simulink model "intSystem"  (R2026a)
settings: Solver=ode3  StopTime=1  FixedStep=xp.Ts
model workspace (MATLAB code in the model file):
  | ip = invParams();
  | wp = windParams();
  | wp = rmfield(wp, {'li_inv','Cp'});   % function handles cannot live on a block
  | xp = intParams();
libraries: fl_lib x17, nesl_utility x15, ee_lib x5, invLib x4, slpidlib x3, windLib x2, simulink x1
settings Model: Creator=khiem  LastModifiedBy=khiem
settings DebuggingCC: AlgebraicLoopMsg=error
settings SimscapeCC: SimscapeLogType=none

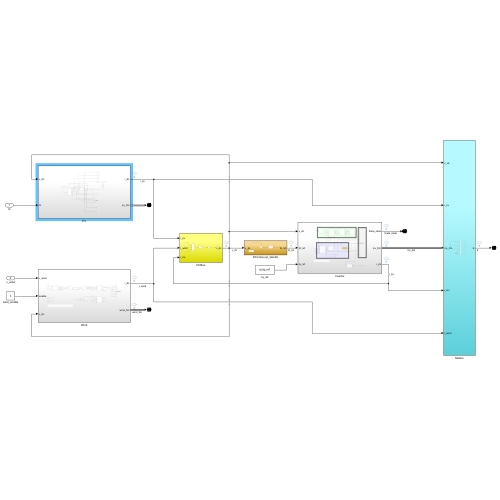
[thumbnail: Simulink's stored preview of the top-level diagram]
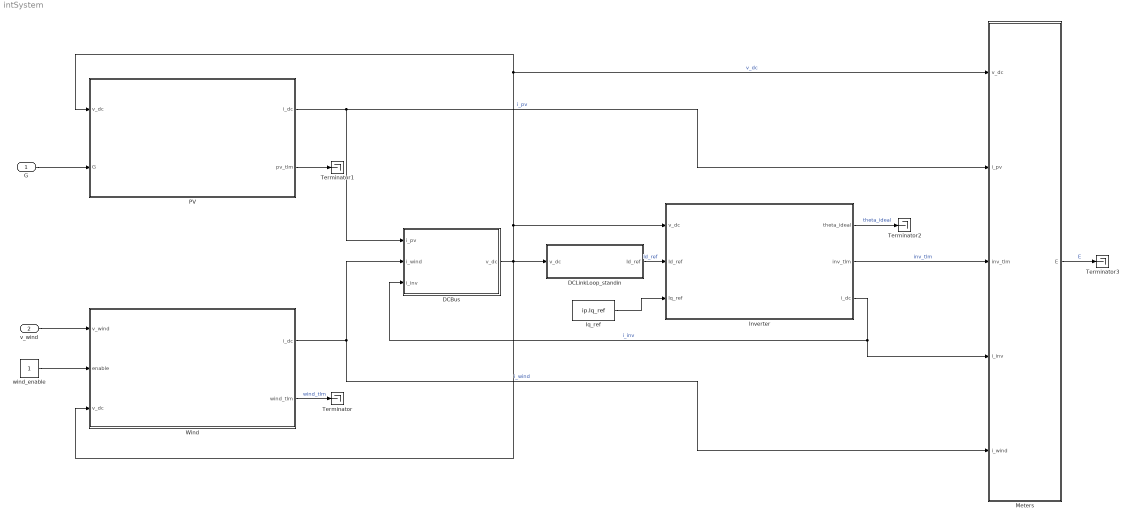
== system intSystem ==
  G : Inport  Interpolate=off
  v_wind : Inport  Port=2  Interpolate=off
  DCBus : Subsystem
  DCLinkLoop_standin : Subsystem
  Inverter : Subsystem
  Iq_ref : Constant  Value=ip.Iq_ref
  Meters : Subsystem
  PV : Subsystem
  Terminator{,1..3} (4 alike) : Terminator
  Wind : Subsystem
  wind_enable : Constant
  wires:
  Inverter/2(inv_tlm) -> Meters/3(inv_tlm)  "inv_tlm"
  G/1 -> PV/2(G)
  v_wind/1 -> Wind/1(v_wind)
  wind_enable/1 -> Wind/2(enable)
  Iq_ref/1 -> Inverter/3(Iq_ref)
  PV/1(i_dc) -> DCBus/1(i_pv), Meters/2(i_pv)  "i_pv"
  Wind/1(i_dc) -> DCBus/2(i_wind), Meters/5(i_wind)  "i_wind"
  Inverter/3(i_dc) -> Meters/4(i_inv), DCBus/3(i_inv)  "i_inv"
  DCBus/1(v_dc) -> Inverter/1(v_dc), Meters/1(v_dc), PV/1(v_dc), DCLinkLoop_standin/1(v_dc), Wind/3(v_dc)  "v_dc"
  DCLinkLoop_standin/1(Id_ref) -> Inverter/2(Id_ref)  "Id_ref"
  Wind/2(wind_tlm) -> Terminator/1  "wind_tlm"
  PV/2(pv_tlm) -> Terminator1/1
  Inverter/1(theta_ideal) -> Terminator2/1  "theta_ideal"
  Meters/1(E) -> Terminator3/1  "E"

== system intSystem/DCBus ==
  i_pv : Inport
  i_wind : Inport  Port=2
  i_inv : Inport  Port=3
  Add : Sum  Inputs=++-
  Gain : Gain  Gain=1/xp.C_bus
  Integrator : Integrator  InitialCondition=xp.Vdc0
  v_dc : Outport
  wires:
  Add/1 -> Gain/1
  Gain/1 -> Integrator/1
  Integrator/1 -> v_dc/1
  i_pv/1 -> Add/1
  i_wind/1 -> Add/2
  i_inv/1 -> Add/3

== system intSystem/DCLinkLoop_standin ==
  v_dc : Inport
  PID Controller : slpidlib/PID Controller  Controller=PI  Form=Parallel  TimeDomain=Discrete-time  UseExternalTs=off  SampleTime=xp.Ts_ctrl  IntegratorMethod=Forward Euler  FilterMethod=Forward Euler  ControllerParametersSource=internal  P=xp.dc.Kp  I=xp.dc.Ki  UseKiTs=off  D=0  UseExternalDerivativeSource=off  N=100  UseFilter=on  TunerSelectOption=Transfer Function Based (PID Tuner App)  InitialConditionSource=internal  InitialConditionForIntegrator=0  InitialConditionForFilter=0  DifferentiatorICPrevScaledInput=0  ExternalReset=none  TrackingMode=off  Kt=1  LimitOutput=on  SatLimitsSource=internal  UpperSaturationLimit=xp.dc.Id_max  LowerSaturationLimit=-xp.dc.Id_max  LinearizeAsGain=on  AntiWindupMode=clamping  Kb=1  LimitIntegrator=off  UpperIntegratorSaturationLimit=inf  LowerIntegratorSaturationLimit=-inf  POutMin=[]  POutMax=[]  IOutMin=[]  IOutMax=[]  DOutMin=[]  DOutMax=[]  NOutMin=[]  NOutMax=[]  SumOutMin=[]  SumOutMax=[]  SaturationOutMin=[]  SaturationOutMax=[]  PParamMin=[]  PParamMax=[]  IParamMin=[]  IParamMax=[]  DParamMin=[]  DParamMax=[]  NParamMin=[]  NParamMax=[]  KbParamMin=[]  KbParamMax=[]  KtParamMin=[]  KtParamMax=[]  KbOutMin=[]  KbOutMax=[]  KtOutMin=[]  KtOutMax=[]  IntegratorOutMin=[]  IntegratorOutMax=[]  FilterOutMin=[]  FilterOutMax=[]  SumI1OutMin=[]  SumI1OutMax=[]  SumI2OutMin=[]  SumI2OutMax=[]  SumI3OutMin=[]  SumI3OutMax=[]  SumI4OutMin=[]  SumI4OutMax=[]  SumDOutMin=[]  SumDOutMax=[]  DifferentiatorOutMin=[]  DifferentiatorOutMax=[]  FilterDiffOutCoefMin=[]  FilterDiffOutCoefMax=[]  ReciprocalOutMin=[]  ReciprocalOutMax=[]  SumDenOutMin=[]  SumDenOutMax=[]  SumNumOutMin=[]  SumNumOutMax=[]  DivideOutMin=[]  DivideOutMax=[]  UdiffTsProdOutMin=[]  UdiffTsProdOutMax=[]  NTsProdOutMin=[]  NTsProdOutMax=[]  UintegralTsProdOutMin=[]  UintegralTsProdOutMax=[]  UngainTsProdOutMin=[]  UngainTsProdOutMax=[]  ClampingZeroOutDataTypeStr=Inherit: Inherit via back propagation  ClampingZeroOutMin=[]  ClampingZeroOutMax=[]  FilterDenConstantOutDataTypeStr=Inherit: Inherit via back propagation  FilterDenConstantOutMin=[]  FilterDenConstantOutMax=[]  PCopyOutDataTypeStr=Inherit: Inherit via back propagation  PCopyOutMin=[]  PCopyOutMax=[]  NCopyOutDataTypeStr=Inherit: Inherit via back propagation  NCopyOutMin=[]  NCopyOutMax=[]  IntegratorContinuousStateAttributes=''  IntegratorStateMustResolveToSignalObject=off  IntegratorRTWStateStorageClass=Auto  FilterContinuousStateAttributes=''  FilterStateMustResolveToSignalObject=off  FilterRTWStateStorageClass=Auto  ParallelPVariant=InternalParameters  IdealPVariant=Disabled  IVariant=InternalParameters  DVariant=Disabled  IntegratorVariant=Discrete  SatVariant=Enabled  AWVariant=DiscClampingParallel  PCopyVariant=Disabled  TRVariant=Disabled  FdbkBlocksVariant=Forward  IdealPFdbkVariant=Disabled  SatFdbkVariant=Disabled  DerivativeFilterVariant=Disabled  NVariant=Disabled  NCopyVariant=Disabled_SignalSpec  FilterICVariant=Disabled  IntegratorICVariant=InternalICs  ExternalResetVariant=Disabled  TRSumVariant=Passthrough  SumFdbkVariant=Disabled  SumVariant=Sum_PI  TsampFilterVariant=InternalTs  TsampNgainVariant=Passthrough  TsampIntegralVariant=Disabled_SignalSpec  ExternalSaturationOutDataTypeStr=Inherit: Same as second input  DerivativeSourceVariant=Disabled  PreIntVariant=InternalPreInt
  Sum : Sum  Inputs=+-
  Vdc_ref : Constant  Value=xp.Vdc_ref
  Id_ref : Outport
  wires:
  v_dc/1 -> Sum/1
  PID Controller/1 -> Id_ref/1
  Sum/1 -> PID Controller/1
  Vdc_ref/1 -> Sum/2

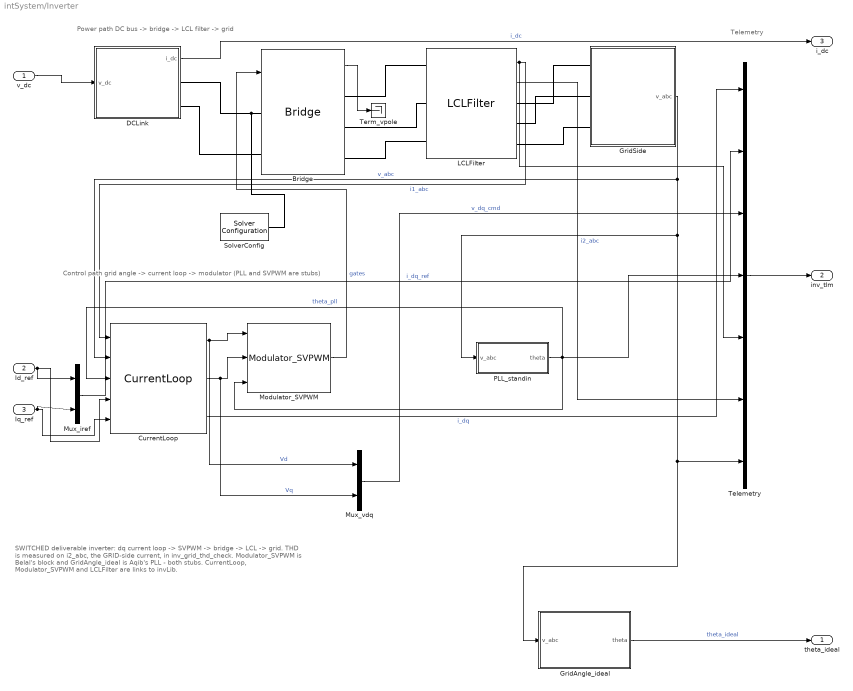
== system intSystem/Inverter ==
  note: SWITCHED deliverable inverter: dq current loop -> SVPWM -> bridge -> LCL -> grid.
      | THD is measured on i2_abc, the GRID-side current, in inv_grid_thd_check.
      | Modulator_SVPWM is Belal's block and GridAngle_ideal is Aqib's PLL - both stubs.
      | CurrentLoop, Modulator_SVPWM and LCLFilter are links to invLib.
  note: Power path DC bus -> bridge -> LCL filter -> grid
  note: Telemetry
  note: Control path grid angle -> current loop -> modulator (PLL and SVPWM are stubs)
  v_dc : Inport
  Id_ref : Inport  Port=2
  Iq_ref : Inport  Port=3
  Bridge : invLib/Bridge  SystemSampleTime=-1  VariantActivationTime=update diagram  EmptyChoice=off  PassThrough=off  PassThroughVariantControl=(default)  EmptyChoiceVariantControl=(default)  AllowFlexibleInterface=on  Latency=0  AutoFrameSizeCalculation=off
  CurrentLoop : invLib/CurrentLoop  SystemSampleTime=-1  VariantActivationTime=update diagram  EmptyChoice=off  PassThrough=off  PassThroughVariantControl=(default)  EmptyChoiceVariantControl=(default)  AllowFlexibleInterface=on  Latency=0  AutoFrameSizeCalculation=off
  DCLink : Subsystem
  GridAngle_ideal : Subsystem
  GridSide : Subsystem
  LCLFilter : invLib/LCLFilter  SystemSampleTime=-1  VariantActivationTime=update diagram  EmptyChoice=off  PassThrough=off  PassThroughVariantControl=(default)  EmptyChoiceVariantControl=(default)  AllowFlexibleInterface=on  Latency=0  AutoFrameSizeCalculation=off
  Modulator_SVPWM : invLib/Modulator_SVPWM  SystemSampleTime=-1  VariantActivationTime=update diagram  EmptyChoice=off  PassThrough=off  PassThroughVariantControl=(default)  EmptyChoiceVariantControl=(default)  AllowFlexibleInterface=on  Latency=0  AutoFrameSizeCalculation=off
  Mux_iref : Mux  Inputs=2
  Mux_vdq : Mux  Inputs=2
  PLL_standin : Subsystem
  SolverConfig : nesl_utility/Solver Configuration  PhysicalDomain=network_engine_domain  SubClassName=solver  LeftPortType=input  RightPortType=generic  Tones=[]  Harmonics=[]  SimulateNoise=off  Profile=off  UseLocalSampling=off  EnableSwitchedLinearOptims=on  FrequencyDomain=off  UseCCode=off  RelTol=0.001  AbsTol=0.001  MinStep=1e-09  ToWorkspace=off  RevertToSquareIcSolve=off  NumHomotopyIterations=100  PhasorMode=off  PhasorModeNumHarmonics=1  ConsistencySolver=NEWTON_XTOL_AFTER_FTOL  CanonicalOrdering=CANONICAL  OptimizeIntermediates=OPTIMIZED  IndexReductionMethod=DerivativeReplacement  DoDC=off  ResidualTolerance=1e-09  ConsistencyTolSource=GLOBAL  ConsistencyAbsTol=0.001  ConsistencyRelTol=0.001  ConsistencyTolFactor=0.001  UseLocalSolver=on  LocalSolverChoice=NE_BACKWARD_EULER_ADVANCER  ResolveIndetEquations=on  FunctionEvalNumThread=1  LocalSolverSampleTime=ip.Ts_power  DoFixedCost=off  MaxNonlinIter=3  MaxModeIter=2  ComputeImpulses=off  ImpulseIterations=2  LinearAlgebra=auto  LinearAlgebraNumThread=0  EquationFormulation=NE_TIME_EF  DelaysMemoryBudget=1024  AutomaticFiltering=on  FilteringTimeConstant=0.001  PartitionStorageMethod=AS_NEEDED  PartitionMemoryBudget=1024  PartitionMethod=ROBUST  MultibodyUseLocalSolver=off  MultibodyLocalSolverChoice=ODE1  MultibodyLocalSolverSampleTime=0.001
  Telemetry : BusCreator  Inputs=7
  Term_vpole : Terminator
  theta_ideal : Outport
  inv_tlm : Outport  Port=2
  i_dc : Outport  Port=3
  wires:
  Bridge/1 -> Term_vpole/1
  GridSide/1(v_abc) -> PLL_standin/1(v_abc), GridAngle_ideal/1(v_abc), Telemetry/7, CurrentLoop/2  "v_abc"
  Mux_iref/1 -> Telemetry/2  "i_dq_ref"
  CurrentLoop/3 -> Telemetry/1  "i_dq"
  CurrentLoop/1 -> Modulator_SVPWM/1, Mux_vdq/1  "Vd"
  CurrentLoop/2 -> Modulator_SVPWM/2, Mux_vdq/2  "Vq"
  Modulator_SVPWM/1 -> Bridge/1  "gates"
  LCLFilter/1 -> CurrentLoop/1, Telemetry/5  "i1_abc"
  Id_ref/1 -> CurrentLoop/4, Mux_iref/1
  Iq_ref/1 -> CurrentLoop/5, Mux_iref/2
  DCLink/1(i_dc) -> i_dc/1  "i_dc"
  Telemetry/1 -> inv_tlm/1
  Mux_vdq/1 -> Telemetry/3  "v_dq_cmd"
  v_dc/1 -> DCLink/1(v_dc)
  LCLFilter/2 -> Telemetry/6  "i2_abc"
  PLL_standin/1(theta) -> CurrentLoop/3, Telemetry/4, Modulator_SVPWM/3  "theta_pll"
  GridAngle_ideal/1(theta) -> theta_ideal/1  "theta_ideal"
  connections:
  SolverConfig/RConn1 -- Bridge/LConn1 -- DCLink/RConn1
  Bridge/RConn3 -- LCLFilter/LConn3
  Bridge/RConn1 -- LCLFilter/LConn1
  LCLFilter/RConn1 -- GridSide/LConn1
  Bridge/RConn2 -- LCLFilter/LConn2
  LCLFilter/RConn3 -- GridSide/LConn3
  DCLink/RConn2 -- Bridge/LConn2
  LCLFilter/RConn2 -- GridSide/LConn2

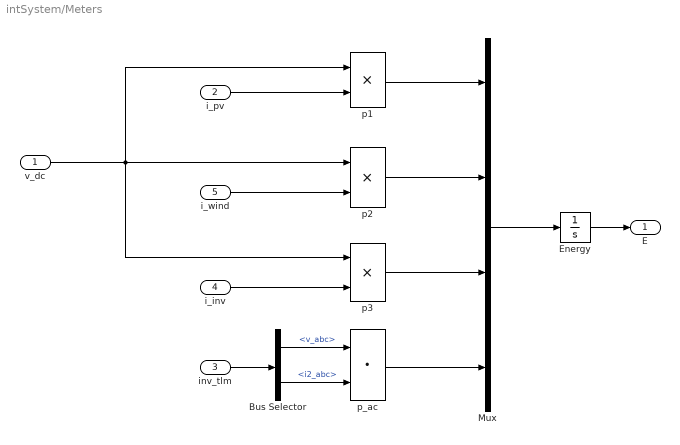
== system intSystem/Meters ==
  v_dc : Inport
  i_pv : Inport  Port=2
  inv_tlm : Inport  Port=3
  i_inv : Inport  Port=4
  i_wind : Inport  Port=5
  Bus Selector : BusSelector  OutputSignals=v_abc,i2_abc
  Energy : Integrator
  Mux : Mux
  p1 : Product
  p2 : Product
  p3 : Product
  p_ac : DotProduct  OutDataTypeStr=Inherit: Inherit via internal rule
  E : Outport
  wires:
  Energy/1 -> E/1
  v_dc/1 -> p3/1, p2/1, p1/1
  i_pv/1 -> p1/2
  i_wind/1 -> p2/2
  i_inv/1 -> p3/2
  p1/1 -> Mux/1
  p2/1 -> Mux/2
  p3/1 -> Mux/3
  inv_tlm/1 -> Bus Selector/1
  Bus Selector/1 -> p_ac/1  "<v_abc>"
  Bus Selector/2 -> p_ac/2  "<i2_abc>"
  p_ac/1 -> Mux/4
  Mux/1 -> Energy/1

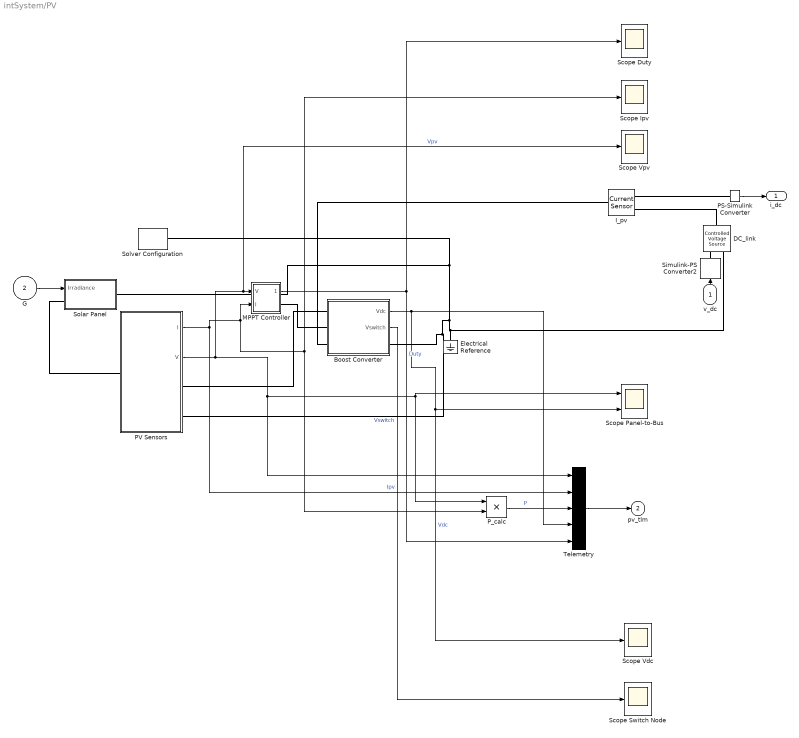
== system intSystem/PV ==
  v_dc : Inport
  G : Inport  Port=2
  Boost Converter : Subsystem
  DC_link : fl_lib/Electrical/Electrical Sources/Controlled Voltage Source
  Electrical Reference : fl_lib/Electrical/Electrical Elements/Electrical Reference
  I_pv : fl_lib/Electrical/Electrical Sensors/Current Sensor
  MPPT Controller : Subsystem
  PS-Simulink Converter : nesl_utility/PS-Simulink Converter  PhysicalDomain=network_engine_domain  SubClassName=ps_output  LeftPortType=input  RightPortType=output  PseudoPeriodic=off  Frequencies=[]  VectorFormat=inherit  Unit=inherit  AffineConversion=off
  PV Sensors : Subsystem
  P_calc : Product
  Scope Duty : Scope
      settings: ActiveDisplayYMinimum=0  ActiveDisplayYMaximum=1
  Scope Ipv : Scope
      settings: ActiveDisplayYMinimum=-14.400000000000034  ActiveDisplayYMaximum=363.59999999999997  DataLoggingVariableName=ScopeData2
  Scope Panel-to-Bus : Scope  NumInputPorts=2
      settings: ActiveDisplayYMinimum=83.437432046539357  ActiveDisplayYMaximum=741.599411880045  DataLoggingVariableName=ScopeData3
  Scope Switch Node : Scope
      settings: ActiveDisplayYMinimum=0  ActiveDisplayYMaximum=800  DataLoggingVariableName=ScopeData4
  Scope Vdc : Scope
      settings: ActiveDisplayYMinimum=551.00007250796614  ActiveDisplayYMaximum=792.77452483583806  DataLoggingVariableName=ScopeData5
  Scope Vpv : Scope
      settings: ActiveDisplayYMinimum=-836.38107028754  ActiveDisplayYMaximum=1247.3439297124605
  Simulink-PS Converter2 : nesl_utility/Simulink-PS Converter  PhysicalDomain=network_engine_domain  SubClassName=ps_input  LeftPortType=input  RightPortType=output  PseudoPeriodic=off  Frequencies=[]  NoiseDistribution=none  NoiseParameters=[]  Unit=1  AffineConversion=off  FilteringAndDerivatives=filter  SimscapeFilterOrder=2  InputFilterTimeConstant=1e-4  UdotUserProvided=0
  Solar Panel : Subsystem  mask(PV Panel){CellTempC=25}
      mask prompts: CellTempC "Cell Temperature (degC)"
      mask help: PV array (5S/48P scaled cell array). Temperature is a per-run parameter, not a live signal -- this Solar Cell block variant has no thermal port (confirmed: no H-port exists), so T_cell cannot vary continuously during one simulation. Set it here before each run.
  Solver Configuration : nesl_utility/Solver Configuration  PhysicalDomain=network_engine_domain  SubClassName=solver  LeftPortType=input  RightPortType=generic  Tones=[]  Harmonics=[]  SimulateNoise=off  Profile=off  UseLocalSampling=off  EnableSwitchedLinearOptims=on  FrequencyDomain=off  UseCCode=off  RelTol=0.001  AbsTol=0.001  MinStep=1e-09  ToWorkspace=off  RevertToSquareIcSolve=off  NumHomotopyIterations=100  PhasorMode=off  PhasorModeNumHarmonics=1  ConsistencySolver=NEWTON_XTOL_AFTER_FTOL  CanonicalOrdering=CANONICAL  OptimizeIntermediates=OPTIMIZED  IndexReductionMethod=DerivativeReplacement  DoDC=off  ResidualTolerance=1e-09  ConsistencyTolSource=GLOBAL  ConsistencyAbsTol=0.001  ConsistencyRelTol=0.001  ConsistencyTolFactor=0.001  UseLocalSolver=on  LocalSolverChoice=NE_BACKWARD_EULER_ADVANCER  ResolveIndetEquations=on  FunctionEvalNumThread=1  LocalSolverSampleTime=xp.Ts  DoFixedCost=off  MaxNonlinIter=3  MaxModeIter=2  ComputeImpulses=off  ImpulseIterations=2  LinearAlgebra=auto  LinearAlgebraNumThread=0  EquationFormulation=NE_TIME_EF  DelaysMemoryBudget=1024  AutomaticFiltering=on  FilteringTimeConstant=0.001  PartitionStorageMethod=AS_NEEDED  PartitionMemoryBudget=1024  PartitionMethod=ROBUST  MultibodyUseLocalSolver=off  MultibodyLocalSolverChoice=ODE1  MultibodyLocalSolverSampleTime=0.001
  Telemetry : BusCreator  Inputs=5
  i_dc : Outport
  pv_tlm : Outport  Port=2
  wires:
  v_dc/1 -> Simulink-PS Converter2/1
  PV Sensors/1(I) -> MPPT Controller/2(I), P_calc/2, Scope Ipv/1, Telemetry/2  "Ipv"
  Boost Converter/2(Vswitch) -> Scope Switch Node/1  "Vswitch"
  MPPT Controller/1(Duty) -> Scope Duty/1, Telemetry/5  "Duty"
  PV Sensors/2(V) -> Telemetry/1, P_calc/1, Scope Panel-to-Bus/1, Scope Vpv/1, MPPT Controller/1(V)  "Vpv"
  G/1 -> Solar Panel/1(Irradiance)
  Boost Converter/1(Vdc) -> Telemetry/4, Scope Vdc/1, Scope Panel-to-Bus/2  "Vdc"
  Telemetry/1 -> pv_tlm/1
  P_calc/1 -> Telemetry/3  "P"
  PS-Simulink Converter/1 -> i_dc/1
  connections:
  PV Sensors/RConn2 -- Boost Converter/RConn1 -- Solver Configuration/RConn1 -- Solar Panel/RConn1 -- DC_link/RConn2 -- Electrical Reference/LConn1
  MPPT Controller/RConn1 -- Boost Converter/LConn2
  PV Sensors/RConn1 -- Boost Converter/LConn1
  Solar Panel/LConn1 -- PV Sensors/LConn1
  Simulink-PS Converter2/RConn1 -- DC_link/RConn1
  Boost Converter/LConn3 -- I_pv/LConn1
  I_pv/RConn2 -- DC_link/LConn1
  I_pv/RConn1 -- PS-Simulink Converter/LConn1

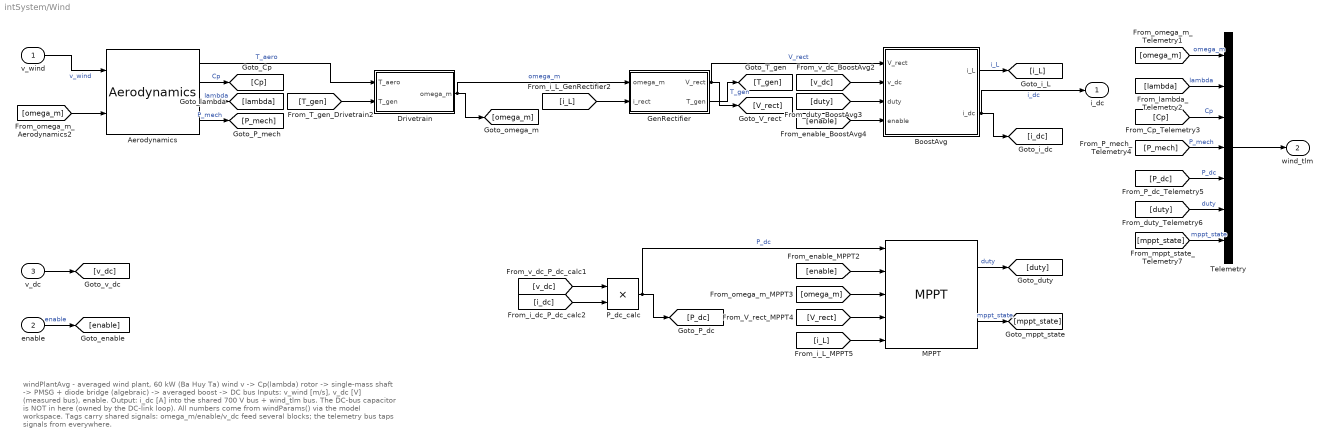
== system intSystem/Wind ==
  note: windPlantAvg - averaged wind plant, 60 kW (Ba Huy Ta)
      | wind v -> Cp(lambda) rotor -> single-mass shaft -> PMSG + diode bridge (algebraic) -> averaged boost -> DC bus
      | Inputs: v_wind [m/s], v_dc [V] (measured bus), enable.  Output: i_dc [A] into the shared 700 V bus + wind_tlm bus.
      | The DC-bus capacitor is NOT in here (owned by the DC-link loop). All numbers come from windParams() via the model workspace.
      | Tags carry shared signals: omega_m/enable/v_dc feed several blocks; the telemetry bus taps signals from everywhere.
  v_wind : Inport
  enable : Inport  Port=2
  v_dc : Inport  Port=3
  Aerodynamics : windLib/Aerodynamics  SystemSampleTime=-1  VariantActivationTime=update diagram  EmptyChoice=off  PassThrough=off  PassThroughVariantControl=(default)  EmptyChoiceVariantControl=(default)  AllowFlexibleInterface=on  Latency=0  AutoFrameSizeCalculation=off
  BoostAvg : Subsystem
  Drivetrain : Subsystem
  GenRectifier : Subsystem
  MPPT : windLib/MPPT  SystemSampleTime=-1  VariantActivationTime=update diagram  EmptyChoice=off  PassThrough=off  PassThroughVariantControl=(default)  EmptyChoiceVariantControl=(default)  AllowFlexibleInterface=on  Latency=0  AutoFrameSizeCalculation=off
  P_dc_calc : Product
  Telemetry : BusCreator  Inputs=7
  i_dc : Outport
  wind_tlm : Outport  Port=2
  wires:
  [omega_m] -> Aerodynamics/2
  [v_dc] -> BoostAvg/2(v_dc)
  [i_dc] -> P_dc_calc/2
  [T_gen] -> Drivetrain/2(T_gen)
  [i_L] -> GenRectifier/2(i_rect)
  Aerodynamics/2 -> [Cp]  "Cp"
  GenRectifier/1(V_rect) -> [V_rect], BoostAvg/1(V_rect)  "V_rect"
  Aerodynamics/4 -> [P_mech]  "P_mech"
  enable/1 -> [enable]  "enable"
  MPPT/1 -> [duty]  "duty"
  Aerodynamics/3 -> [lambda]  "lambda"
  Drivetrain/1(omega_m) -> [omega_m], GenRectifier/1(omega_m)  "omega_m"
  [mppt_state] -> Telemetry/7  "mppt_state"
  Aerodynamics/1 -> Drivetrain/1(T_aero)  "T_aero"
  [P_mech] -> Telemetry/4  "P_mech"
  [v_dc] -> P_dc_calc/1
  [duty] -> BoostAvg/3(duty)
  GenRectifier/2(T_gen) -> [T_gen]  "T_gen"
  v_dc/1 -> [v_dc]
  [enable] -> BoostAvg/4(enable)
  Telemetry/1 -> wind_tlm/1
  [duty] -> Telemetry/6  "duty"
  [enable] -> MPPT/2
  [omega_m] -> MPPT/3
  [Cp] -> Telemetry/3  "Cp"
  [omega_m] -> Telemetry/1  "omega_m"
  [lambda] -> Telemetry/2  "lambda"
  [V_rect] -> MPPT/4
  P_dc_calc/1 -> [P_dc], MPPT/1  "P_dc"
  [i_L] -> MPPT/5
  MPPT/2 -> [mppt_state]  "mppt_state"
  [P_dc] -> Telemetry/5  "P_dc"
  BoostAvg/2(i_dc) -> [i_dc], i_dc/1  "i_dc"
  v_wind/1 -> Aerodynamics/1  "v_wind"
  BoostAvg/1(i_L) -> [i_L]  "i_L"

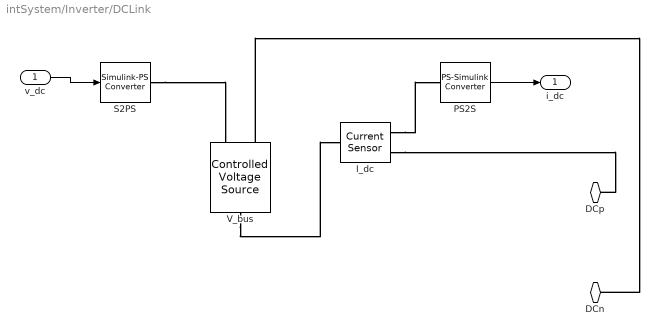
== system intSystem/Inverter/DCLink ==
  v_dc : Inport
  I_dc : fl_lib/Electrical/Electrical Sensors/Current Sensor
  PS2S : nesl_utility/PS-Simulink Converter  PhysicalDomain=network_engine_domain  SubClassName=ps_output  LeftPortType=input  RightPortType=output  PseudoPeriodic=off  Frequencies=[]  VectorFormat=inherit  Unit=inherit  AffineConversion=off
  S2PS : nesl_utility/Simulink-PS Converter  PhysicalDomain=network_engine_domain  SubClassName=ps_input  LeftPortType=input  RightPortType=output  PseudoPeriodic=off  Frequencies=[]  NoiseDistribution=none  NoiseParameters=[]  Unit=1  AffineConversion=off  FilteringAndDerivatives=provide  SimscapeFilterOrder=1  InputFilterTimeConstant=0.001  UdotUserProvided=0
  V_bus : fl_lib/Electrical/Electrical Sources/Controlled Voltage Source
  DCp : PMIOPort  Side=Right
  DCn : PMIOPort  Port=2  Side=Right
  i_dc : Outport
  wires:
  v_dc/1 -> S2PS/1
  PS2S/1 -> i_dc/1
  connections:
  S2PS/RConn1 -- V_bus/RConn1
  V_bus/LConn1 -- I_dc/LConn1
  I_dc/RConn2 -- DCp/RConn1
  V_bus/RConn2 -- DCn/RConn1
  I_dc/RConn1 -- PS2S/LConn1

== system intSystem/Inverter/GridAngle_ideal ==
  v_abc : Inport
  grid_angle : MATLAB Function  TreatAsAtomicUnit=on
  sample_theta : UnitDelay  SampleTime=ip.Ts_ctrl
  theta : Outport
  wires:
  v_abc/1 -> grid_angle/1(v_abc)
  grid_angle/1(theta) -> sample_theta/1
  sample_theta/1 -> theta/1

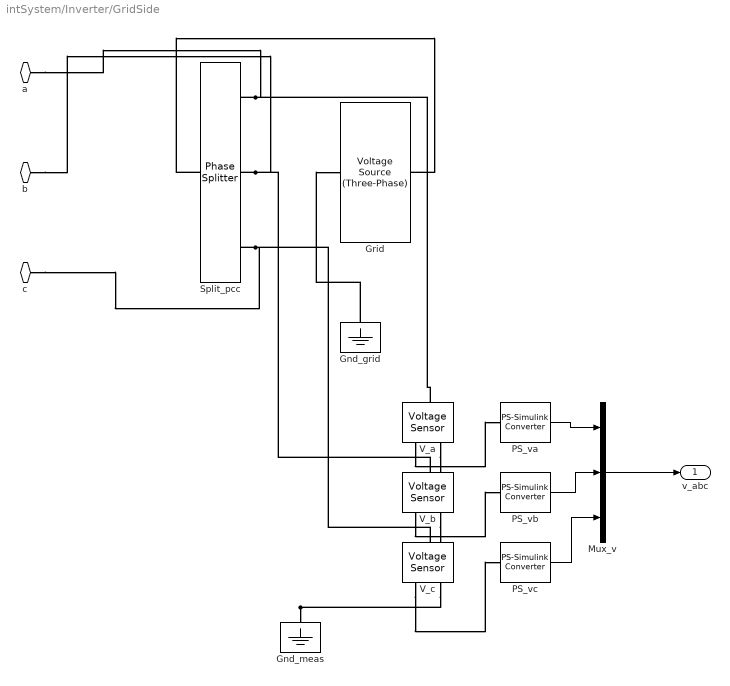
== system intSystem/Inverter/GridSide ==
  Gnd_grid : fl_lib/Electrical/Electrical Elements/Electrical Reference
  Gnd_meas : fl_lib/Electrical/Electrical Elements/Electrical Reference
  Grid : ee_lib/Sources/Voltage Source (Three-Phase)  vline_rms=ip.V_ll V  shift=0 deg  freq=ip.f_grid Hz  impedance_option=ip.grid_Z_opt  SShortCircuit=ip.S_sc A*V  XR=ip.grid_XR  R=0.01 Ohm  L=3.97e-4 H  harmonic_option=0  harmonic_orders=[5, 7, 11, 13]  harmonic_ratios=[.1, .1, .1, .1]  G_parasitic=0 1/Ohm  I_specify=off  I_priority=None  I=[0, 0, 0] A  I_nominal_specify=off  I_nominal_value=1  I_nominal_unit=A
  Mux_v : Mux  Inputs=3
  PS_va : nesl_utility/PS-Simulink Converter  PhysicalDomain=network_engine_domain  SubClassName=ps_output  LeftPortType=input  RightPortType=output  PseudoPeriodic=off  Frequencies=[]  VectorFormat=inherit  Unit=inherit  AffineConversion=off
  PS_vb : nesl_utility/PS-Simulink Converter  PhysicalDomain=network_engine_domain  SubClassName=ps_output  LeftPortType=input  RightPortType=output  PseudoPeriodic=off  Frequencies=[]  VectorFormat=inherit  Unit=inherit  AffineConversion=off
  PS_vc : nesl_utility/PS-Simulink Converter  PhysicalDomain=network_engine_domain  SubClassName=ps_output  LeftPortType=input  RightPortType=output  PseudoPeriodic=off  Frequencies=[]  VectorFormat=inherit  Unit=inherit  AffineConversion=off
  Split_pcc : ee_lib/Connectors & References/Phase Splitter
  V_a : fl_lib/Electrical/Electrical Sensors/Voltage Sensor
  V_b : fl_lib/Electrical/Electrical Sensors/Voltage Sensor
  V_c : fl_lib/Electrical/Electrical Sensors/Voltage Sensor
  a : PMIOPort  Side=Left
  b : PMIOPort  Port=2  Side=Left
  c : PMIOPort  Port=3  Side=Left
  v_abc : Outport
  wires:
  PS_va/1 -> Mux_v/1
  PS_vb/1 -> Mux_v/2
  PS_vc/1 -> Mux_v/3
  Mux_v/1 -> v_abc/1
  connections:
  Split_pcc/LConn1 -- Grid/RConn1
  Gnd_grid/LConn1 -- Grid/LConn1
  Split_pcc/RConn1 -- a/RConn1 -- V_a/LConn1
  V_a/RConn2 -- V_b/RConn2 -- Gnd_meas/LConn1 -- V_c/RConn2
  V_a/RConn1 -- PS_va/LConn1
  Split_pcc/RConn2 -- b/RConn1 -- V_b/LConn1
  V_b/RConn1 -- PS_vb/LConn1
  Split_pcc/RConn3 -- c/RConn1 -- V_c/LConn1
  V_c/RConn1 -- PS_vc/LConn1

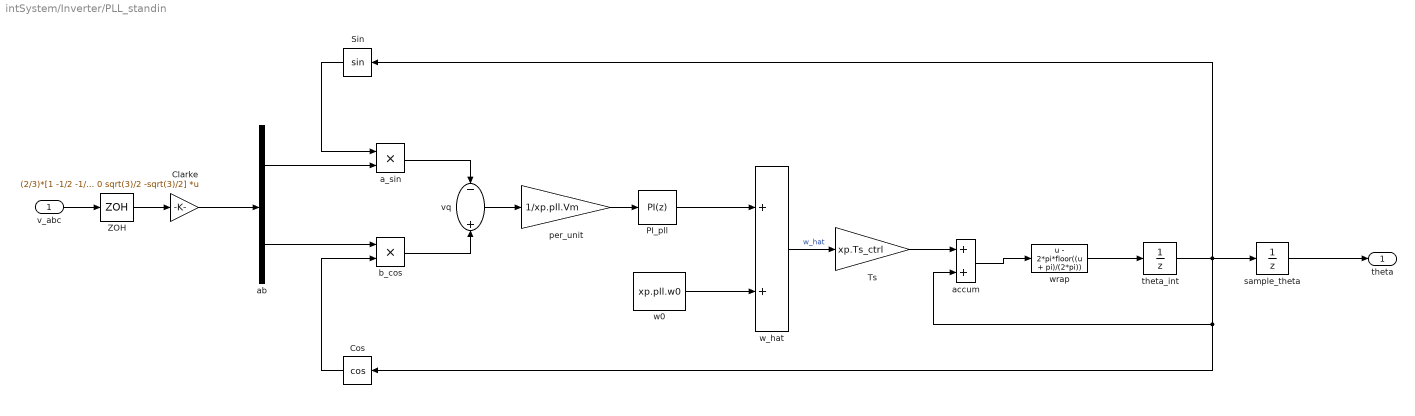
== system intSystem/Inverter/PLL_standin ==
  v_abc : Inport
  " Ts" : Gain  Gain=xp.Ts_ctrl
  " w_hat" : Sum
  Clarke : Gain  Gain=(2/3)*[1 -1/2 -1/2; 0 sqrt(3)/2 -sqrt(3)/2]  Multiplication=Matrix(K*u)
  Cos : Trigonometry  Operator=cos
  PI_pll : slpidlib/PID Controller  Controller=PI  Form=Parallel  TimeDomain=Discrete-time  UseExternalTs=off  SampleTime=xp.Ts_ctrl  IntegratorMethod=Forward Euler  FilterMethod=Forward Euler  ControllerParametersSource=internal  P=xp.pll.Kp  I=xp.pll.Ki  UseKiTs=off  D=0  UseExternalDerivativeSource=off  N=100  UseFilter=on  TunerSelectOption=Transfer Function Based (PID Tuner App)  InitialConditionSource=internal  InitialConditionForIntegrator=0  InitialConditionForFilter=0  DifferentiatorICPrevScaledInput=0  ExternalReset=none  TrackingMode=off  Kt=1  LimitOutput=off  SatLimitsSource=internal  UpperSaturationLimit=inf  LowerSaturationLimit=-inf  LinearizeAsGain=on  AntiWindupMode=none  Kb=1  LimitIntegrator=off  UpperIntegratorSaturationLimit=inf  LowerIntegratorSaturationLimit=-inf  POutMin=[]  POutMax=[]  IOutMin=[]  IOutMax=[]  DOutMin=[]  DOutMax=[]  NOutMin=[]  NOutMax=[]  SumOutMin=[]  SumOutMax=[]  SaturationOutMin=[]  SaturationOutMax=[]  PParamMin=[]  PParamMax=[]  IParamMin=[]  IParamMax=[]  DParamMin=[]  DParamMax=[]  NParamMin=[]  NParamMax=[]  KbParamMin=[]  KbParamMax=[]  KtParamMin=[]  KtParamMax=[]  KbOutMin=[]  KbOutMax=[]  KtOutMin=[]  KtOutMax=[]  IntegratorOutMin=[]  IntegratorOutMax=[]  FilterOutMin=[]  FilterOutMax=[]  SumI1OutMin=[]  SumI1OutMax=[]  SumI2OutMin=[]  SumI2OutMax=[]  SumI3OutMin=[]  SumI3OutMax=[]  SumI4OutMin=[]  SumI4OutMax=[]  SumDOutMin=[]  SumDOutMax=[]  DifferentiatorOutMin=[]  DifferentiatorOutMax=[]  FilterDiffOutCoefMin=[]  FilterDiffOutCoefMax=[]  ReciprocalOutMin=[]  ReciprocalOutMax=[]  SumDenOutMin=[]  SumDenOutMax=[]  SumNumOutMin=[]  SumNumOutMax=[]  DivideOutMin=[]  DivideOutMax=[]  UdiffTsProdOutMin=[]  UdiffTsProdOutMax=[]  NTsProdOutMin=[]  NTsProdOutMax=[]  UintegralTsProdOutMin=[]  UintegralTsProdOutMax=[]  UngainTsProdOutMin=[]  UngainTsProdOutMax=[]  ClampingZeroOutDataTypeStr=Inherit: Inherit via back propagation  ClampingZeroOutMin=[]  ClampingZeroOutMax=[]  FilterDenConstantOutDataTypeStr=Inherit: Inherit via back propagation  FilterDenConstantOutMin=[]  FilterDenConstantOutMax=[]  PCopyOutDataTypeStr=Inherit: Inherit via back propagation  PCopyOutMin=[]  PCopyOutMax=[]  NCopyOutDataTypeStr=Inherit: Inherit via back propagation  NCopyOutMin=[]  NCopyOutMax=[]  IntegratorContinuousStateAttributes=''  IntegratorStateMustResolveToSignalObject=off  IntegratorRTWStateStorageClass=Auto  FilterContinuousStateAttributes=''  FilterStateMustResolveToSignalObject=off  FilterRTWStateStorageClass=Auto  ParallelPVariant=InternalParameters  IdealPVariant=Disabled  IVariant=InternalParameters  DVariant=Disabled  IntegratorVariant=Discrete  SatVariant=Disabled  AWVariant=Passthrough  PCopyVariant=Disabled  TRVariant=Disabled  FdbkBlocksVariant=Forward  IdealPFdbkVariant=Disabled  SatFdbkVariant=Disabled  DerivativeFilterVariant=Disabled  NVariant=Disabled  NCopyVariant=Disabled_SignalSpec  FilterICVariant=Disabled  IntegratorICVariant=InternalICs  ExternalResetVariant=Disabled  TRSumVariant=Passthrough  SumFdbkVariant=Disabled  SumVariant=Sum_PI  TsampFilterVariant=InternalTs  TsampNgainVariant=Passthrough  TsampIntegralVariant=Disabled_SignalSpec  ExternalSaturationOutDataTypeStr=Inherit: Same as second input  DerivativeSourceVariant=Disabled  PreIntVariant=InternalPreInt
  Sin : Trigonometry
  ZOH : ZeroOrderHold  SampleTime=xp.Ts_ctrl
  a_sin : Product
  ab : Demux  Outputs=2
  accum : Sum
  b_cos : Product
  per_unit : Gain  Gain=1/xp.pll.Vm
  sample_theta : UnitDelay  InitialCondition=xp.pll.theta0  SampleTime=xp.Ts_ctrl
  theta_int : UnitDelay  InitialCondition=xp.pll.theta0  SampleTime=xp.Ts_ctrl
  vq : Sum  Inputs=-+
  w0 : Constant  Value=xp.pll.w0
  wrap : Fcn  Expr=u - 2*pi*floor((u + pi)/(2*pi))
  theta : Outport
  wires:
  v_abc/1 -> ZOH/1
  ZOH/1 -> Clarke/1
  Clarke/1 -> ab/1
  ab/1 -> a_sin/2
  ab/2 -> b_cos/1
  a_sin/1 -> vq/1
  b_cos/1 -> vq/2
  vq/1 -> per_unit/1
  per_unit/1 -> PI_pll/1
  PI_pll/1 -> " w_hat"/1
  wrap/1 -> theta_int/1
  theta_int/1 -> Sin/1, sample_theta/1, Cos/1, accum/2
  w0/1 -> " w_hat"/2
  " w_hat"/1 -> " Ts"/1  "w_hat"
  " Ts"/1 -> accum/1
  accum/1 -> wrap/1
  sample_theta/1 -> theta/1
  Cos/1 -> b_cos/2
  Sin/1 -> a_sin/1

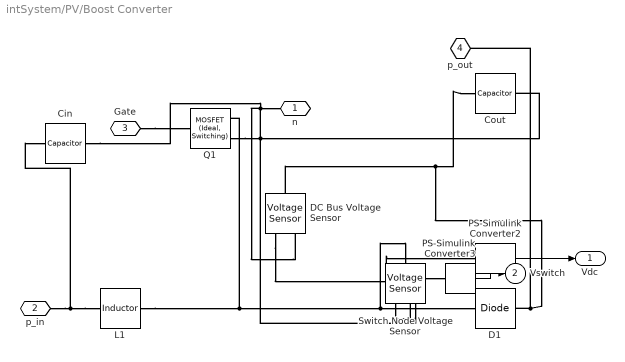
== system intSystem/PV/Boost Converter ==
  Cin : fl_lib/Electrical/Electrical Elements/Capacitor  c=1000e-6 F  r=1e-6 Ohm  g=0 1/Ohm  i_specify=off  i_priority=None  i=0 A  i_nominal_specify=off  i_nominal_value=1  i_nominal_unit=A  v_specify=off  v_priority=None  v=0 V  v_nominal_specify=off  v_nominal_value=1  v_nominal_unit=V  vc_specify=off  vc_priority=High  vc=0 V  vc_nominal_specify=off  vc_nominal_value=1  vc_nominal_unit=V
  Cout : fl_lib/Electrical/Electrical Elements/Capacitor  c=1200e-6 F  r=1e-6 Ohm  g=0 1/Ohm  i_specify=off  i_priority=None  i=0 A  i_nominal_specify=off  i_nominal_value=1  i_nominal_unit=A  v_specify=off  v_priority=High  v=xp.Vdc0 V  v_nominal_specify=off  v_nominal_value=1  v_nominal_unit=V  vc_specify=on  vc_priority=High  vc=xp.Vdc0 V  vc_nominal_specify=off  vc_nominal_value=1  vc_nominal_unit=V
  D1 : ee_lib/Semiconductors & Converters/Diode  ModelType=ee.enum.diode.modelType.pwl  TableType=ee.enum.diode.tableType.IfMat  IfMat=[.07, .12, .19, 1.75, 4.24, 7.32, 11.2; .16, .3, .72, 2.14, 5.02, 8.35, 13.12] A  VfMat=[.9, 1.15, 1.25, 1.5, 1.75, 2.17, 2.6, 2.85; .58, .68, .75, 1.1, 1.38, 1.77, 2.27, 2.7] V  TjVec=[25, 125] degC  VfVec=[.5, .7, .9, 1.3, 1.7, 2.1, 2.5] V  IfVec=[.1, .2, .5, 1, 2, 4, 7, 10] A  IrMat=[1e-06, 2e-06, 5e-06, 1e-05, 2.5e-05, 5e-05, .0001; 2e-06, 5e-06, 1e-05, 4e-05, 8e-05, .0002, .0005] A  VrMat=[10, 100, 200, 250, 300, 325, 350; 10, 70, 160, 220, 270, 300, 320] V  VrVec=[10, 20, 40, 50, 70, 80, 100] V  IrVec=[1e-06, 2e-06, 5e-06, 1e-05, 2e-05, 5e-05, .0001] A  Vf=0.6 V  Ron=0.3 Ohm  Goff=1e-8 S  prmExp=ee.enum.diode.expParam.useTwo  I12=[.0137, .545] A  V12=[.6, .7] V  RS=0 Ohm  Tmeas=298.15 K  IS=1e-12 A  ec=1  I1=0.0137 A  V1=0.6 V  N_series=1  N_parallel=1  ZenerEnable=false  Rz=0.3 Ohm  BV=30 V  C_param=ee.enum.diode.capParam.fixed  CJ=0 pF  CJ0=5 pF  Vvec=[.1, 10, 100] V  Cvec=[3.5, 1, .4] pF  VJ=1 V  Mgrad=0.5  FC=0.5  Q_param=ee.enum.diode.recoveryParam.off  iRM=-7.15 A  iF=4 A  didt=-750 A/us  trr_factor=3  trr=115 ns  Qrr=150 nA*s  Vr=-600 V  Ls=150 nH  Erec=0.03 J  TT=50 ns  tau=100 ns  T_param=ee.enum.diode.temperatureParam.off  Tdevice=298.15 K  I1_T2=0.245 A  V1_T2=0.5 V  IS_T2=1.25e-7 A  Tmeas2=125 degC  XTI_param=ee.enum.diode.xtiParam.pn  XTI=3  EG_param=ee.enum.diode.egapParam.material_si  EG=1.11 eV  dBVdT=0 V/K  enable_fault_input=simscape.enum.onoff.off  i_specify=off  i_priority=None  i=0 A  i_nominal_specify=off  i_nominal_value=1  i_nominal_unit=A  v_specify=off  v_priority=None  v=0 V  v_nominal_specify=off  v_nominal_value=1  v_nominal_unit=V  v_capacitor_specify=off  v_capacitor_priority=None  v_capacitor=0 V  v_capacitor_nominal_specify=off  v_capacitor_nominal_value=1  v_capacitor_nominal_unit=V  Qj_specify=off  Qj_priority=High  Qj=0 C  Qj_nominal_specify=off  Qj_nominal_value=1  Qj_nominal_unit=C  i_diode_specify=off  i_diode_priority=None  i_diode=0 A  i_diode_nominal_specify=off  i_diode_nominal_value=1  i_diode_nominal_unit=A  v_diode_specify=off  v_diode_priority=None  v_diode=0 V  v_diode_nominal_specify=off  v_diode_nominal_value=1  v_diode_nominal_unit=V  i_capacitor_specify=off  i_capacitor_priority=None  i_capacitor=0 A  i_capacitor_nominal_specify=off  i_capacitor_nominal_value=1  i_capacitor_nominal_unit=A  fidelity_level=ee.enum.diode.fidelity.includeChargeDyn  rec_loss_model=ee.enum.diode.reverseRecoveryModelTabulateUpTo3D.fixed  ErecVal=0 J  scaleWithIandV=true  ErecMat=zeros(2, 3) J  ErecMat3D=zeros(2, 3, 2) J  TjrecVec=[298.15, 398.15] K  IfrecVec=[.1, 1, 10] A  IrecVal=10 A  VrecVal=10 V  VrecVec=[0, 100] V  tFilter=1 / 1000 / 100 s  thermal_network_parameterization=ee.enum.thermalNetworkTopology.junctionCase  Rth=[0, 10] K/W  Rth_Cauer=[1, 3, 10] K/W  Rth_Foster=[.08, .14, .22, .16] K/W  thermal_mass_parameterization=ee.enum.thermalNetwork.timeconstant  thermal_mass=[0, 1] J/K  thermal_mass_Cauer=[.1, .3, 1] J/K  thermal_mass_Foster=[.001, .005, .05, .5] J/K  thermal_time_constant=[0, 10] s  thermal_time_constant_Cauer=[1, 3, 10] s  thermal_time_constant_Foster=[7e-05, .0007, .01, .08] s  thermal_mass_initial_temperatures=[25, 25] degC  thermal_mass_initial_temperatures_Cauer=[25, 25, 25] degC  junction_thermal_mass=0.01 J/K  Tvec_initial_Foster=[25, 25, 25, 25] degC  no_thermal_network=0  junction_temperature_specify=off  junction_temperature_priority=None  junction_temperature=25 degC  junction_temperature_nominal_specify=off  junction_temperature_nominal_value=1  junction_temperature_nominal_unit=degC
  DC Bus Voltage Sensor : fl_lib/Electrical/Electrical Sensors/Voltage Sensor
  L1 : fl_lib/Electrical/Electrical Elements/Inductor  l=500e-6 H  r=0 Ohm  g=1e-9 1/Ohm  i_specify=off  i_priority=None  i=0 A  i_nominal_specify=off  i_nominal_value=1  i_nominal_unit=A  v_specify=off  v_priority=None  v=0 V  v_nominal_specify=off  v_nominal_value=1  v_nominal_unit=V  i_L_specify=off  i_L_priority=High  i_L=0 A  i_L_nominal_specify=off  i_L_nominal_value=1  i_L_nominal_unit=A
  PS-Simulink Converter2 : nesl_utility/PS-Simulink Converter  PhysicalDomain=network_engine_domain  SubClassName=ps_output  LeftPortType=input  RightPortType=output  PseudoPeriodic=off  Frequencies=[]  VectorFormat=inherit  Unit=inherit  AffineConversion=off
  PS-Simulink Converter3 : nesl_utility/PS-Simulink Converter  PhysicalDomain=network_engine_domain  SubClassName=ps_output  LeftPortType=input  RightPortType=output  PseudoPeriodic=off  Frequencies=[]  VectorFormat=inherit  Unit=inherit  AffineConversion=off
  Q1 : ee_lib/Semiconductors & Converters/MOSFET (Ideal, Switching)  port_option=ee.enum.controlport.ps  Rds=0.01 Ohm  Goff=1e-6 1/Ohm  Vth=2 V  diode_param=ee.enum.semiconductors.protectionDiode.nodynamics  diode_Vf=0.8 V  diode_Ron=0.001 Ohm  diode_Goff=1e-5 1/Ohm  diode_C=50e-9 F  diode_iRM=-235 A  diode_iF=300 A  diode_idot=-50 A/us  diode_trr_param=ee.enum.converters.diodeReverseParam.trr_factor  diode_trr_factor=3  diode_trr=15 us  diode_Qrr=1500 s*uA  ids_specify=off  ids_priority=None  ids=0 A  ids_nominal_specify=off  ids_nominal_value=1  ids_nominal_unit=A  vds_specify=off  vds_priority=None  vds=0 V  vds_nominal_specify=off  vds_nominal_value=1  vds_nominal_unit=V  vgs_specify=off  vgs_priority=None  vgs=0 V  vgs_nominal_specify=off  vgs_nominal_value=1  vgs_nominal_unit=V  thermal_loss_option=ee.enum.converters.thermalLossOption.constantvalues  Von_data=[0, 1.8, 3.2, 6, 10, 16; 0, 2, 5.5, 9.5, 15, 25] V  Tj=[298.15, 448.15] K  Iout_data=[0, 20, 40, 60, 80, 100] A  tabulateWithVds=false  Eon_data=[0, 55.04, 124.57, 235.53, 362.12; 0, 71.25, 161.25, 304.88, 468.75] * 1e-6 J  Eoff_data=[0, 18, 30, 56.1, 76.5; 0, 22.5, 37.5, 70.13, 95.63] * 1e-6 J  Eon_data_3D=[zeros(2, 5, 3)] J  Eoff_data_3D=[zeros(2, 5, 3)] J  Tj_loss=[298.15, 448.15] K  Iout_data_loss=[0, 10, 20, 30, 40] A  Vds_loss=[0, 150, 300] V  Eon_scalar=22.86e-3 J  Eoff_scalar=17.14e-3 J  Voff=300 V  Iout_scalar=600 A  useCurrentFromPreviousCycle=false  useVoltageFromPreviousCycle=false  diodeModelType=ee.enum.converters.diodeModelType.pwl  diodeTableType=ee.enum.diode.tableType.IfMat  diode_ReverseIVType=ee.enum.diode.diodeReverseIV.constant  diode_IfMat=[.07, .12, .19, 1.75, 4.24, 7.32, 11.2; .16, .3, .72, 2.14, 4.02, 6.35, 9.12] A  diode_VfMat=[.9, 1.15, 1.25, 1.5, 1.75, 2.17, 2.6, 2.85; .58, .68, .75, 1.1, 1.38, 1.77, 2.27, 2.7] V  diode_TjVec=[25, 125] degC  diode_VfVec=[.5, .7, .9, 1.3, 1.7, 2.1, 2.5] V  diode_IfVec=[.1, .2, .5, 1, 2, 4, 7, 10] A  diode_IrMat=[1e-06, 2e-06, 5e-06, 1e-05, 2.5e-05, 5e-05, .0001; 2e-06, 5e-06, 1e-05, 4e-05, 8e-05, .0002, .0005] A  diode_VrMat=[10, 100, 200, 250, 300, 325, 350; 10, 70, 160, 220, 270, 300, 320] V  diode_VrVec=[10, 20, 40, 50, 70, 80, 100] V  diode_IrVec=[1e-06, 2e-06, 5e-06, 1e-05, 2e-05, 5e-05, .0001] A  diode_Vr=-600 V  diode_Ls=150 nH  diode_Erec=0.03 J  diode_rec_loss_model=ee.enum.diode.reverseRecoveryModelTabulateUpTo3D.fixed  diode_ErecVal=0 J  diode_scaleWithIandV=true  diode_ErecMat=zeros(2, 3) J  diodeErecMat3D=zeros(2, 3, 2) J  diode_TjrecVec=[298.15, 398.15] K  diode_IfrecVec=[.1, 1, 10] A  diodeVrecVec=[0, 100] V  diode_IrecVal=10 A  diode_VrecVal=10 V  diode_tFilter=1 / 1000 / 100 s  separateThermalPortForDiode=false  thermal_network_parameterization=ee.enum.thermalNetworkTopology.external  Rth=[.03, .2] K/W  Rth_Cauer=[.03, .1, .2] K/W  Rth_Foster=[.08, .14, .22, .16] K/W  thermal_mass_parameterization=ee.enum.thermalNetwork.timeconstant  thermal_mass=[3, 25] J/K  thermal_mass_Cauer=[3, 10, 25] J/K  thermal_mass_Foster=[.001, .005, .05, .5] J/K  thermal_time_constant=[.1, 5] s  thermal_time_constant_Cauer=[.1, 1, 5] s  thermal_time_constant_Foster=[7e-05, .0007, .01, .08] s  thermal_mass_initial_temperatures=[25, 25] degC  thermal_mass_initial_temperatures_Cauer=[25, 25, 25] degC  junction_thermal_mass=0.1 J/K  Tvec_initial_Foster=[25, 25, 25, 25] degC  RthDiode=[.03, .2] K/W  RthCauerDiode=[.03, .1, .2] K/W  RthFosterDiode=[.03, .2] K/W  thermalMassDiode=[3, 25] J/K  thermalMassCauerDiode=[3, 10, 25] J/K  thermalMassFosterDiode=[33, 50] J/K  thermalTauDiode=[.1, 5] s  thermalTauCauerDiode=[.1, 1, 5] s  thermalTauFosterDiode=[1, 10] s  thermalMassInitTempDiode=[25, 25] degC  thermalMassInitTempCauerDiode=[25, 25, 25] degC  junctionthermalMassDiode=0.1 J/K  TVecInitialFosterDiode=[25, 25, 25, 25] degC  no_thermal_network=ee.enum.enable.no  mosfet_junction_temperature_specify=off  mosfet_junction_temperature_priority=None  mosfet_junction_temperature=25 degC  mosfet_junction_temperature_nominal_specify=off  mosfet_junction_temperature_nominal_value=1  mosfet_junction_temperature_nominal_unit=degC  diode_junction_temperature_specify=off  diode_junction_temperature_priority=None  diode_junction_temperature=25 degC  diode_junction_temperature_nominal_specify=off  diode_junction_temperature_nominal_value=1  diode_junction_temperature_nominal_unit=degC  Qj_specify=off  Qj_priority=None  Qj=0 W  Qj_nominal_specify=off  Qj_nominal_value=1  Qj_nominal_unit=W  accumulatedSwitchingLosses_specify=off  accumulatedSwitchingLosses_priority=None  accumulatedSwitchingLosses=0 J
  Switch Node Voltage Sensor : fl_lib/Electrical/Electrical Sensors/Voltage Sensor
  n : PMIOPort  Side=Right
  p_in : PMIOPort  Port=2  Side=Left
  Gate : PMIOPort  Port=3  Side=Left
  p_out : PMIOPort  Port=4  Side=Left
  Vdc : Outport
  Vswitch : Outport  Port=2
  wires:
  PS-Simulink Converter2/1 -> Vdc/1
  PS-Simulink Converter3/1 -> Vswitch/1
  connections:
  L1/LConn1 -- p_in/RConn1 -- Cin/LConn1
  Gate/RConn1 -- Q1/LConn1
  DC Bus Voltage Sensor/RConn1 -- PS-Simulink Converter2/LConn1
  Cout/RConn1 -- n/RConn1 -- Cin/RConn1 -- DC Bus Voltage Sensor/RConn2 -- Switch Node Voltage Sensor/RConn2 -- Q1/RConn2
  L1/RConn1 -- Switch Node Voltage Sensor/LConn1 -- D1/LConn1 -- Q1/RConn1
  Cout/LConn1 -- DC Bus Voltage Sensor/LConn1 -- D1/RConn1 -- p_out/RConn1
  Switch Node Voltage Sensor/RConn1 -- PS-Simulink Converter3/LConn1

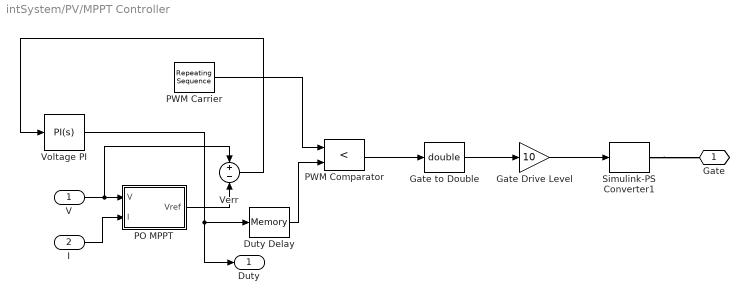
== system intSystem/PV/MPPT Controller ==
  V : Inport
  I : Inport  Port=2
  Duty Delay : Memory  InitialCondition=0.5
  Gate Drive Level : Gain  Gain=10
  Gate to Double : DataTypeConversion  OutDataTypeStr=double  SaturateOnIntegerOverflow=off  RndMeth=Floor
  PO MPPT : MATLAB Function  TreatAsAtomicUnit=on  SystemSampleTime=0.01
  PWM Carrier : simulink/Sources/Repeating Sequence  rep_seq_t=[0 1e-4]  rep_seq_y=[0 1]
  PWM Comparator : RelationalOperator  Operator=<  OutDataTypeStr=boolean  RndMeth=Simplest  InputSameDT=off
  Simulink-PS Converter1 : nesl_utility/Simulink-PS Converter  PhysicalDomain=network_engine_domain  SubClassName=ps_input  LeftPortType=input  RightPortType=output  PseudoPeriodic=off  Frequencies=[]  NoiseDistribution=none  NoiseParameters=[]  Unit=1  AffineConversion=off  FilteringAndDerivatives=provide  SimscapeFilterOrder=1  InputFilterTimeConstant=0.001  UdotUserProvided=0
  Verr : Sum  Inputs=+-
  Voltage PI : slpidlib/PID Controller  Controller=PI  Form=Parallel  TimeDomain=Continuous-time  UseExternalTs=off  SampleTime=-1  IntegratorMethod=Forward Euler  FilterMethod=Forward Euler  ControllerParametersSource=internal  P=0.0008  I=0.03  UseKiTs=off  D=0  UseExternalDerivativeSource=off  N=100  UseFilter=on  TunerSelectOption=Transfer Function Based (PID Tuner App)  InitialConditionSource=internal  InitialConditionForIntegrator=0.5  InitialConditionForFilter=0  DifferentiatorICPrevScaledInput=0  ExternalReset=none  TrackingMode=off  Kt=1  LimitOutput=on  SatLimitsSource=internal  UpperSaturationLimit=0.95  LowerSaturationLimit=0.05  LinearizeAsGain=on  AntiWindupMode=back-calculation  Kb=1  LimitIntegrator=off  UpperIntegratorSaturationLimit=inf  LowerIntegratorSaturationLimit=-inf  POutMin=[]  POutMax=[]  IOutMin=[]  IOutMax=[]  DOutMin=[]  DOutMax=[]  NOutMin=[]  NOutMax=[]  SumOutMin=[]  SumOutMax=[]  SaturationOutMin=[]  SaturationOutMax=[]  PParamMin=[]  PParamMax=[]  IParamMin=[]  IParamMax=[]  DParamMin=[]  DParamMax=[]  NParamMin=[]  NParamMax=[]  KbParamMin=[]  KbParamMax=[]  KtParamMin=[]  KtParamMax=[]  KbOutMin=[]  KbOutMax=[]  KtOutMin=[]  KtOutMax=[]  IntegratorOutMin=[]  IntegratorOutMax=[]  FilterOutMin=[]  FilterOutMax=[]  SumI1OutMin=[]  SumI1OutMax=[]  SumI2OutMin=[]  SumI2OutMax=[]  SumI3OutMin=[]  SumI3OutMax=[]  SumI4OutMin=[]  SumI4OutMax=[]  SumDOutMin=[]  SumDOutMax=[]  DifferentiatorOutMin=[]  DifferentiatorOutMax=[]  FilterDiffOutCoefMin=[]  FilterDiffOutCoefMax=[]  ReciprocalOutMin=[]  ReciprocalOutMax=[]  SumDenOutMin=[]  SumDenOutMax=[]  SumNumOutMin=[]  SumNumOutMax=[]  DivideOutMin=[]  DivideOutMax=[]  UdiffTsProdOutMin=[]  UdiffTsProdOutMax=[]  NTsProdOutMin=[]  NTsProdOutMax=[]  UintegralTsProdOutMin=[]  UintegralTsProdOutMax=[]  UngainTsProdOutMin=[]  UngainTsProdOutMax=[]  ClampingZeroOutDataTypeStr=Inherit: Inherit via back propagation  ClampingZeroOutMin=[]  ClampingZeroOutMax=[]  FilterDenConstantOutDataTypeStr=Inherit: Inherit via back propagation  FilterDenConstantOutMin=[]  FilterDenConstantOutMax=[]  PCopyOutDataTypeStr=Inherit: Inherit via back propagation  PCopyOutMin=[]  PCopyOutMax=[]  NCopyOutDataTypeStr=Inherit: Inherit via back propagation  NCopyOutMin=[]  NCopyOutMax=[]  IntegratorContinuousStateAttributes=''  IntegratorStateMustResolveToSignalObject=off  IntegratorRTWStateStorageClass=Auto  FilterContinuousStateAttributes=''  FilterStateMustResolveToSignalObject=off  FilterRTWStateStorageClass=Auto  ParallelPVariant=InternalParameters  IdealPVariant=Disabled  IVariant=InternalParameters  DVariant=Disabled  IntegratorVariant=Continuous  SatVariant=Enabled  AWVariant=BackCalculation  PCopyVariant=Disabled  TRVariant=Disabled  FdbkBlocksVariant=Forward  IdealPFdbkVariant=Disabled  SatFdbkVariant=Disabled  DerivativeFilterVariant=Disabled  NVariant=Disabled  NCopyVariant=Disabled_SignalSpec  FilterICVariant=Disabled  IntegratorICVariant=InternalICs  ExternalResetVariant=Disabled  TRSumVariant=Passthrough  SumFdbkVariant=Disabled  SumVariant=Sum_PI  TsampFilterVariant=InternalTs  TsampNgainVariant=Passthrough  TsampIntegralVariant=Disabled_SignalSpec  ExternalSaturationOutDataTypeStr=Inherit: Same as second input  DerivativeSourceVariant=Disabled  PreIntVariant=InternalPreInt
  Gate : PMIOPort  Side=Right
  Duty : Outport
  wires:
  Duty Delay/1 -> PWM Comparator/2
  V/1 -> PO MPPT/1(V), Verr/1
  PWM Comparator/1 -> Gate to Double/1
  I/1 -> PO MPPT/2(I)
  Gate to Double/1 -> Gate Drive Level/1
  PWM Carrier/1 -> PWM Comparator/1
  Gate Drive Level/1 -> Simulink-PS Converter1/1
  PO MPPT/1(Vref) -> Verr/2
  Verr/1 -> Voltage PI/1
  Voltage PI/1 -> Duty Delay/1, Duty/1
  connections:
  Simulink-PS Converter1/RConn1 -- Gate/RConn1

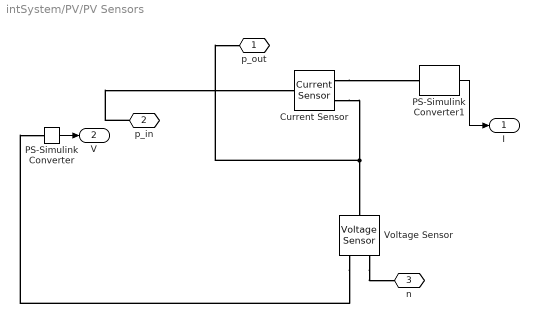
== system intSystem/PV/PV Sensors ==
  Current Sensor : fl_lib/Electrical/Electrical Sensors/Current Sensor
  PS-Simulink Converter : nesl_utility/PS-Simulink Converter  PhysicalDomain=network_engine_domain  SubClassName=ps_output  LeftPortType=input  RightPortType=output  PseudoPeriodic=off  Frequencies=[]  VectorFormat=inherit  Unit=inherit  AffineConversion=off
  PS-Simulink Converter1 : nesl_utility/PS-Simulink Converter  PhysicalDomain=network_engine_domain  SubClassName=ps_output  LeftPortType=input  RightPortType=output  PseudoPeriodic=off  Frequencies=[]  VectorFormat=inherit  Unit=inherit  AffineConversion=off
  Voltage Sensor : fl_lib/Electrical/Electrical Sensors/Voltage Sensor
  p_out : PMIOPort  Side=Right
  p_in : PMIOPort  Port=2  Side=Left
  n : PMIOPort  Port=3  Side=Right
  I : Outport
  V : Outport  Port=2
  wires:
  PS-Simulink Converter1/1 -> I/1
  PS-Simulink Converter/1 -> V/1
  connections:
  Current Sensor/RConn2 -- p_out/RConn1 -- Voltage Sensor/LConn1
  Voltage Sensor/RConn2 -- n/RConn1
  Current Sensor/RConn1 -- PS-Simulink Converter1/LConn1
  Voltage Sensor/RConn1 -- PS-Simulink Converter/LConn1
  p_in/RConn1 -- Current Sensor/LConn1

== system intSystem/PV/Solar Panel ==
  Irradiance : Inport
  Simulink-PS Converter : nesl_utility/Simulink-PS Converter  PhysicalDomain=network_engine_domain  SubClassName=ps_input  LeftPortType=input  RightPortType=output  PseudoPeriodic=off  Frequencies=[]  NoiseDistribution=none  NoiseParameters=[]  Unit=1  AffineConversion=off  FilteringAndDerivatives=provide  SimscapeFilterOrder=1  InputFilterTimeConstant=0.001  UdotUserProvided=0
  Solar Cell : ee_lib/Sources/Solar Cell  prm=ee.enum.sources.solar_cell_prm.datasheet  Isc=7.34 A  Voc=0.6 V  Is=1e-6 A  Is2=0 A  Iph=7.34 A  Ir0=1000 W/m^2  ec=1.5  N2=2  Rs=0.003 Ohm  Rp=4.1 Ohm  N_series=723  N_parallel=48  TIPH1=0 1/K  EG=1.11 eV  TXIS1=3  TXIS2=3  TRS1=0  TRP1=0  Tmeas=25 degC  TFIXED=CellTempC degC  thermal_mass=100 J/K  initial_temperature=25 degC
  p : PMIOPort  Side=Left
  n : PMIOPort  Port=2  Side=Right
  wires:
  Irradiance/1 -> Simulink-PS Converter/1
  connections:
  Simulink-PS Converter/RConn1 -- Solar Cell/LConn1
  n/RConn1 -- Solar Cell/RConn1
  Solar Cell/LConn2 -- p/RConn1

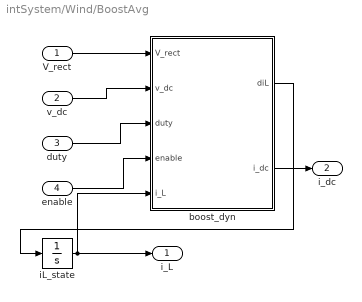
== system intSystem/Wind/BoostAvg ==
  V_rect : Inport
  v_dc : Inport  Port=2
  duty : Inport  Port=3
  enable : Inport  Port=4
  boost_dyn : MATLAB Function  TreatAsAtomicUnit=on
  iL_state : Integrator  InitialCondition=wp.iL_init  LimitOutput=on  LowerSaturationLimit=0
  i_L : Outport
  i_dc : Outport  Port=2
  wires:
  boost_dyn/1(diL) -> iL_state/1
  enable/1 -> boost_dyn/4(enable)
  iL_state/1 -> i_L/1, boost_dyn/5(i_L)
  duty/1 -> boost_dyn/3(duty)
  v_dc/1 -> boost_dyn/2(v_dc)
  boost_dyn/2(i_dc) -> i_dc/1
  V_rect/1 -> boost_dyn/1(V_rect)

== system intSystem/Wind/Drivetrain ==
  T_aero : Inport
  T_gen : Inport  Port=2
  T_net : Sum  Inputs=+--
  damping_B : Gain  Gain=wp.B
  inv_J : Gain  Gain=1/wp.J
  omega_state : Integrator  InitialCondition=wp.w_init  LimitOutput=on  LowerSaturationLimit=0.1
  omega_m : Outport
  wires:
  T_net/1 -> inv_J/1
  damping_B/1 -> T_net/3
  T_gen/1 -> T_net/2
  T_aero/1 -> T_net/1
  inv_J/1 -> omega_state/1
  omega_state/1 -> damping_B/1, omega_m/1

== system intSystem/Wind/GenRectifier ==
  omega_m : Inport
  i_rect : Inport  Port=2
  genrect_fcn : MATLAB Function  TreatAsAtomicUnit=on
  V_rect : Outport
  T_gen : Outport  Port=2
  wires:
  genrect_fcn/2(T_gen) -> T_gen/1
  genrect_fcn/1(V_rect) -> V_rect/1
  i_rect/1 -> genrect_fcn/2(i_rect)
  omega_m/1 -> genrect_fcn/1(omega_m)

== matlab function intSystem/Inverter/GridAngle_ideal/grid_angle ==
  data: v_abc input; theta output
function theta = grid_angle(v_abc)
%#codegen
% Grid voltage angle straight off the Clarke transform. Not a PLL: no loop,
% no filter, no dynamics - which is the point. Aqib's SRF-PLL replaces it,
% and its lag then shows up as a difference against this baseline.
v_al = (2/3)*(v_abc(1) - 0.5*v_abc(2) - 0.5*v_abc(3));
v_be = (2/3)*(sqrt(3)/2)*(v_abc(2) - v_abc(3));
theta = atan2(v_be, v_al);

== matlab function intSystem/PV/MPPT Controller/PO MPPT ==
  data: V input; Vref output; I input
function Vref = po_mppt(V, I)
% Perturb & Observe MPPT (voltage-reference mode).
% Perturbs a panel-voltage setpoint Vref to maximize power P=V*I.
% An outer PI loop then regulates the panel to this Vref by setting duty.
persistent Vref_state Pprev dir
if isempty(Vref_state)
    Vref_state = 360;   % start near expected MPP (V)
    Pprev = 0;
    dir = -1;           % initial search direction
end

dV   = 0.5;             % perturbation step (V)
Vmin = 150;
Vmax = 420;

P = V * I;
if P < Pprev
    dir = -dir;         % power dropped -> reverse direction
end
Vref_state = Vref_state + dir*dV;
Vref_state = min(max(Vref_state, Vmin), Vmax);
Pprev = P;
Vref = Vref_state;

== matlab function intSystem/Wind/BoostAvg/boost_dyn ==
  data: V_rect input; diL output; v_dc input; duty input; enable input; i_L input; i_dc output; wp parameter
function [diL, i_dc] = boost_dyn(V_rect, v_dc, duty, enable, i_L, wp)
%#codegen
% State-space averaged (switching-function) boost converter.
% One state, the inductor current; the switching ripple is deliberately not
% represented - that is what the switched variant is for.

% Duty limits belong to the plant, not the controller: the converter cannot
% exceed them no matter what the MPPT asks for.
d = min(max(duty, wp.d_min), wp.duty_max);
if enable <= 0.5
    d = 0;
end

i = max(i_L, 0);
diL = (V_rect - (1 - d)*v_dc - wp.R_L*i)/wp.L_boost;

% Unidirectional: the boost diode cannot pull current back out of the bus, so
% the current sticks at zero rather than reversing (discontinuous conduction).
if i <= 0 && diL < 0
    diL = 0;
end

% Current delivered to the shared 700 V DC bus.
i_dc = (1 - d)*i;
if enable <= 0.5
    i_dc = 0;
end
end

== matlab function intSystem/Wind/GenRectifier/genrect_fcn ==
  data: omega_m input; V_rect output; i_rect input; T_gen output; wp parameter
function [V_rect, T_gen] = genrect_fcn(omega_m, i_rect, wp)
%#codegen
% PMSG + 3-phase uncontrolled diode bridge, collapsed to its averaged DC form.
%
% The open-circuit relation V_dc = 1.35*V_ll is only the starting point. The
% loading terms below are what stop the bridge behaving like an ideal source -
% without them the MPPT has nothing to hunt against and the result flatters.

w = max(omega_m, 0.1);
i = max(i_rect,  0);        % a diode bridge conducts one way only

w_e  = wp.p*w;                    % electrical rad/s
E_pk = w_e*wp.lam_pm;             % per-phase peak back-EMF
V_ll = E_pk*sqrt(3)/sqrt(2);      % line-to-line rms
V_oc = 1.35*V_ll;                 % ideal 6-pulse rectified voltage

V_rect = V_oc ...
         - (3/pi)*w_e*wp.Ls*i ...    % commutation overlap (source inductance)
         - 2*wp.Rs*i ...             % two phases conducting in series
         - wp.V_f;                   % two diode forward drops
V_rect = max(V_rect, 0);

% Shaft torque must account for ALL power leaving the machine, including the
% losses above - otherwise the drivetrain gets energy for free.
P_gen = V_rect*i + 2*wp.Rs*i^2 + wp.V_f*i;
T_gen = P_gen/w;
end
